simulink model "Linearization2"  (R2022a)
settings: Solver=VariableStepAuto  StartTime=0.0  StopTime=10.0  RelTol=1e-3
undefined symbols (not defined in the file): Aactuator, ac, AeroCoeff, ControlAllocation, DUmax, DUmin, EngineTable, F, fcs, ft, g, hground, IC, kg, LandingGear, Light, LPmethod, m, MIL, Mode_deflection_aileron, Mode_deflection_elevator, Mode_deflection_rudder, Mode_deflection_TVC_y, Mode_deflection_TVC_z, N, Ninv_2nozzle, Ninv_no_nozzle, PIController, s, Sensor, slug, state0, sysID_DAQ, sysID_OBES, Umax_2nozzle, Umax_no_nozzle, Umin_2nozzle, Umin_no_nozzle, WMM2020
libraries: aerolibconvert2 x19, slpidlib x6, simulink x6, sharedutil x4, aerolibatmos2 x3, aerolibwind2 x3, aerolibbdyn x3, aerolibgravity2 x2, sharedtransform x1
(part 3 of 9)

== system Linearization2/F-16 Vehicle Systems Model/Vehicle/Aerodynamics ==
  note: TODO: 這全部源自PlantData(物理系統)，不用感測器
  note: TODO: 這攻角、速度 來自感測器、AeroData System
  note: X
      | Y
      | Z
      | L
      | M
      | N
  note: 攻角 $\alpha$ 限制 -20 ~ 90度
      | 側滑角 $\beta$ 限制 -30 ~ 30 度
      | 馬赫數限制 0.1 ~ 0.6 度
  fcs_cmd : Inport
  " SB (deg)" : Inport  Port=2
  In Bus Element7 : Inport  Port=3  PortName=EnvData  Element=Pressure
  In Bus Element8 : Inport  Port=3  PortName=EnvData  Element=AirDensity
  In Bus Element9 : Inport  Port=3  PortName=EnvData  Element=qbar
  In Bus Element : Inport  Port=4  PortName=PlantData  Element=p
  In Bus Element1 : Inport  Port=4  PortName=PlantData  Element=q
  In Bus Element2 : Inport  Port=4  PortName=PlantData  Element=r
  In Bus Element3 : Inport  Port=4  PortName=PlantData  Element=alpha
  In Bus Element10 : Inport  Port=4  PortName=PlantData  Element=alpha
  In Bus Element4 : Inport  Port=4  PortName=PlantData  Element=beta
  In Bus Element6 : Inport  Port=4  PortName=PlantData  Element=Vt
  In Bus Element5 : Inport  Port=4  PortName=PlantData  Element=Vt
  Aerofynamic Coefficients : Subsystem
  AirframeActuators (no roll off) : Subsystem
  Angle Conversion1 : aerolibconvert2/Angle Conversion  IU=rad  OU=deg
  Angle Conversion2 : aerolibconvert2/Angle Conversion  IU=rad  OU=deg
  Angle Conversion3 : aerolibconvert2/Angle Conversion  Commented=on  IU=rad  OU=deg
  Bus Creator : BusCreator  Inputs=7
  Bus Selector : BusSelector  OutputSignals=right Aileron_deg,left Aileron_deg,right Elevator_deg,left Elevator_deg,Rudder_deg,LEF_deg
  Bus Selector1 : BusSelector  OutputSignals=right Aileron_deg,left Aileron_deg,right Elevator_deg,left Elevator_deg,Rudder_deg,LEF_deg
  Bus Selector2 : BusSelector  Commented=on  OutputSignals=LEF_deg
  Cbar(ft)1 : Constant  Value=ac.cbar
  Goto2 : Goto  Commented=on  GotoTag=LEF_deg
  Ground : Ground
  Leading Edge Flap : Subsystem  Commented=on
  Mux1 : Mux  Inputs=3
  Mux2 : Mux
  Product{6,9..14} (7 alike) : Product
  Sref(ft^2) : Constant  Value=ac.S
  Terminator{,1..3} (4 alike) : Terminator
  Velocity Conversion : aerolibconvert2/Velocity Conversion  Commented=on  IU=ft/s  OU=m/s
  b(ft)1 : Constant  Value=ac.b
  FM : Outport
  Bus Element Out : Outport  Port=2  PortName=ActSensor_Out
  wires:
  " SB (deg)"/1 -> Aerofynamic Coefficients/9(SB (deg)), Bus Creator/7  "SB_deg"
  In Bus Element1/1 -> Aerofynamic Coefficients/12(q)
  In Bus Element/1 -> Aerofynamic Coefficients/11(p)
  Angle Conversion2/1 -> Aerofynamic Coefficients/2(beta (deg))
  Angle Conversion1/1 -> Aerofynamic Coefficients/1(alpha (deg))
  In Bus Element2/1 -> Aerofynamic Coefficients/13(r)
  Ground/1 -> Aerofynamic Coefficients/15(h_AGL), Aerofynamic Coefficients/14(GearAngle)
  Mux1/1 -> Product9/2
  [qbar_S] -> Product9/1
  Aerofynamic Coefficients/6(Cn_T) -> Product14/2
  Aerofynamic Coefficients/5(Cm_T) -> Product12/2
  [qbar_S_cbar] -> Product12/1  "qbar_S_cbar"
  Aerofynamic Coefficients/4(Cl_T) -> Product13/2
  [qbar_S_b] -> Product13/1, Product14/1  "qbar_S_b"
  Aerofynamic Coefficients/1(CX_T) -> Mux1/1
  Aerofynamic Coefficients/2(CY_T) -> Mux1/2
  Aerofynamic Coefficients/3(CZ_T) -> Mux1/3
  Product13/1 -> Mux2/2
  Product12/1 -> Mux2/3
  Product14/1 -> Mux2/4
  Product9/1 -> Mux2/1
  Mux2/1 -> FM/1
  Sref(ft^2)/1 -> Product6/2
  b(ft)1/1 -> Product11/2  "b"
  Product11/1 -> [qbar_S_b]
  Product10/1 -> [qbar_S_cbar]
  Cbar(ft)1/1 -> Product10/2  "cbar"
  In Bus Element9/1 -> Product6/1  "qbar"
  Product6/1 -> Product11/1, Product10/1, [qbar_S]  "qbar_S"
  Leading Edge Flap/2(ActPositions) -> Goto2/1
  Velocity Conversion/1 -> Leading Edge Flap/1(vt (m/s))  "vt (m/s)"
  In Bus Element6/1 -> Aerofynamic Coefficients/10(vt (ft/s))
  In Bus Element8/1 -> Terminator1/1
  In Bus Element7/1 -> Terminator2/1
  AirframeActuators (no roll off)/1(ActPositions) -> Bus Selector/1
  fcs_cmd/1 -> AirframeActuators (no roll off)/1(fcs_cmd)
  In Bus Element3/1 -> Angle Conversion1/1
  In Bus Element4/1 -> Angle Conversion2/1
  In Bus Element5/1 -> Terminator/1  "vt (ft/s)"
  AirframeActuators (no roll off)/2(ActSensor_Out) -> Bus Selector1/1
  Bus Creator/1 -> Bus Element Out/1
  In Bus Element10/1 -> Terminator3/1
  Angle Conversion3/1 -> Leading Edge Flap/4(alpha (deg))
  Leading Edge Flap/1(ActSensor_Out) -> Bus Selector2/1
  Bus Selector1/1 -> Bus Creator/1  "<right Aileron_deg>"
  Bus Selector1/2 -> Bus Creator/2  "<left Aileron_deg>"
  Bus Selector1/3 -> Bus Creator/3  "<right Elevator_deg>"
  Bus Selector1/4 -> Bus Creator/4  "<left Elevator_deg>"
  Bus Selector1/5 -> Bus Creator/5  "<Rudder_deg>"
  Bus Selector1/6 -> Bus Creator/6  "<LEF_deg>"
  Bus Selector/1 -> Aerofynamic Coefficients/3(right alieron (deg))  "<right Aileron_deg>"
  Bus Selector/2 -> Aerofynamic Coefficients/4(left aileron (deg))  "<left Aileron_deg>"
  Bus Selector/3 -> Aerofynamic Coefficients/5(right elevator (deg))  "<right Elevator_deg>"
  Bus Selector/4 -> Aerofynamic Coefficients/6(left elevator (deg))  "<left Elevator_deg>"
  Bus Selector/5 -> Aerofynamic Coefficients/7(rudder (deg))  "<Rudder_deg>"
  Bus Selector/6 -> Aerofynamic Coefficients/8(LEF (deg))  "<LEF_deg>"

== system Linearization2/F-16 Vehicle Systems Model/Vehicle/Gravity Force ==
  note: 轉成行向量(column vector)
  note: 註：重力不會對飛機產生力矩，
      | 因為重力永遠作用在飛機重心上，
      | 力臂=0，所以力矩=0
  DCM_be : Inport
  In Bus Element : Inport  Port=2  PortName=EnvData  Element=g
  Gravity in Earth Axis : Gain  Gain=ac.m
  Reshape : Reshape  OutputDimensionality=Column vector (2-D)
  To Body Axes : Product  Multiplication=Matrix(*)
  Fgrav : Outport
  wires:
  In Bus Element/1 -> Gravity in Earth Axis/1
  To Body Axes/1 -> Fgrav/1
  DCM_be/1 -> To Body Axes/1
  Gravity in Earth Axis/1 -> Reshape/1
  Reshape/1 -> To Body Axes/2

== system Linearization2/F-16 Vehicle Systems Model/Vehicle/LandingGear GroundReaction ==
  note: 定義：
      | 慣性座標+Z軸朝上
      | 體座標+Z軸朝下
  note: 詹庭宇:
      | 此起落架模組源自MATLAB Simulink Example:HL-20
      | 我有做
      | 1.正負號的訂正
      | 2.拿掉/忽略輪胎側向力
  note: 詹庭宇:拿掉/忽略輪胎側向力模型，Fy=0
  LG_cmd : Inport
  In Bus Element4 : Inport  Port=2  PortName=EnvData  Element=hground
  In Bus Element5 : Inport  Port=2  PortName=EnvData  Element=hground
  In Bus Element6 : Inport  Port=2  PortName=EnvData  Element=hground
  In Bus Element3 : Inport  Port=3  PortName=PlantData
  In Bus Element1 : Inport  Port=3  PortName=PlantData
  In Bus Element2 : Inport  Port=3  PortName=PlantData
  Enable : EnablePort
  Demux : Demux  Outputs=3
  L Main Gear Geometry Forces and Moments : Subsystem  TreatAsAtomicUnit=on
  LeftMain : Selector  NumberOfDimensions=2  InputPortWidth=3  IndexOptions=Select all,Index vector (dialog)  Indices=-1,1  OutputSizes=1
  Nose : Selector  NumberOfDimensions=2  InputPortWidth=3  IndexOptions=Select all,Index vector (dialog)  Indices=-1,3  OutputSizes=1
  Nose Gear Geometry Forces and Moments : Subsystem  TreatAsAtomicUnit=on
  Pos_full_extend_ft Rows are X,Y,Z;cols are Left,Right,Nose gear Measured from CG in fts : Constant  Value=[-1.8405,-1.8405,9.9132 ; -3.8753,3.8753,0 ; 5.9161,5.9161, 6.2905]
  R Main Gear Geometry Forces and Moments : Subsystem  TreatAsAtomicUnit=on
  RightMain : Selector  NumberOfDimensions=2  InputPortWidth=3  IndexOptions=Select all,Index vector (dialog)  Indices=-1,2  OutputSizes=1
  Sum2 : Sum  Inputs=+++  InputSameDT=on  SaturateOnIntegerOverflow=on  OutDataTypeStr=Inherit: Same as first input
  FM : Outport
  Out Bus Element3 : Outport  Port=2  VectorParamsAs1DForOutWhenUnconnected=off  PortName=LGData  Element=Nose_WOW
  Out Bus Element4 : Outport  Port=2  VectorParamsAs1DForOutWhenUnconnected=off  PortName=LGData  Element=Nose_GearCmprs
  Out Bus Element5 : Outport  Port=2  VectorParamsAs1DForOutWhenUnconnected=off  PortName=LGData  Element=Nose_LG_down
  Out Bus Element6 : Outport  Port=2  VectorParamsAs1DForOutWhenUnconnected=off  PortName=LGData  Element=LeftMain_WOW
  Out Bus Element7 : Outport  Port=2  VectorParamsAs1DForOutWhenUnconnected=off  PortName=LGData  Element=LeftMain_GearCmprs
  Out Bus Element8 : Outport  Port=2  VectorParamsAs1DForOutWhenUnconnected=off  PortName=LGData  Element=LeftMain_LG_down
  Out Bus Element9 : Outport  Port=2  VectorParamsAs1DForOutWhenUnconnected=off  PortName=LGData  Element=RightMain_WOW
  Out Bus Element10 : Outport  Port=2  VectorParamsAs1DForOutWhenUnconnected=off  PortName=LGData  Element=RightMain_GearCmprs
  Out Bus Element11 : Outport  Port=2  VectorParamsAs1DForOutWhenUnconnected=off  PortName=LGData  Element=RightMain_LG_down
  wires:
  In Bus Element4/1 -> L Main Gear Geometry Forces and Moments/1(ground_z_ft)
  In Bus Element3/1 -> L Main Gear Geometry Forces and Moments/2(plant)
  In Bus Element1/1 -> R Main Gear Geometry Forces and Moments/2(plant)
  In Bus Element2/1 -> Nose Gear Geometry Forces and Moments/2(plant)
  R Main Gear Geometry Forces and Moments/1(FM) -> Sum2/2
  L Main Gear Geometry Forces and Moments/1(FM) -> Sum2/1
  R Main Gear Geometry Forces and Moments/3(GearCmprs) -> Out Bus Element10/1
  R Main Gear Geometry Forces and Moments/2(WOW) -> Out Bus Element9/1
  L Main Gear Geometry Forces and Moments/2(WOW) -> Out Bus Element6/1
  L Main Gear Geometry Forces and Moments/3(GearCmprs) -> Out Bus Element7/1
  RightMain/1 -> R Main Gear Geometry Forces and Moments/3(GearLoc)
  Nose/1 -> Nose Gear Geometry Forces and Moments/3(GearLoc)
  Pos_full_extend_ft Rows are X,Y,Z;cols are Left,Right,Nose gear Measured from CG in fts/1 -> LeftMain/1, Nose/1, RightMain/1
  Nose Gear Geometry Forces and Moments/1(FM) -> Sum2/3
  Nose Gear Geometry Forces and Moments/2(WOW) -> Out Bus Element3/1
  Nose Gear Geometry Forces and Moments/3(GearCmprs) -> Out Bus Element4/1
  Sum2/1 -> FM/1
  LeftMain/1 -> L Main Gear Geometry Forces and Moments/3(GearLoc)
  LG_cmd/1 -> Demux/1
  Demux/1 -> Out Bus Element5/1
  Demux/2 -> Out Bus Element11/1
  Demux/3 -> Out Bus Element8/1
  In Bus Element5/1 -> R Main Gear Geometry Forces and Moments/1(ground_z_ft)
  In Bus Element6/1 -> Nose Gear Geometry Forces and Moments/1(ground_z_ft)

== system Linearization2/F-16 Vehicle Systems Model/Vehicle/Propulsion ==
  note: 繞"固定座標旋轉"旋轉(外在旋轉extrinsic rotation)
  note: Thrust Vector Nozzle Module 向量噴嘴模組
  note: Commands_TVC_rY_pitch_deg
      | Commands_TVC_rZ_yaw_deg
      | Commands_TVC_lY_pitch_deg
      | Commands_TVC_lZ_yaw_deg
  note: Inlet 進氣道
  note: 高度限制 0 ~ 50000 ft
      | 馬赫數限制 0 ~ 1 馬赫
  Bus Element In2 : Inport  PortName=fadec_cmd
  In Bus Element3 : Inport  PortName=fadec_cmd  Element=thrust
  In Bus Element1 : Inport  Port=2  PortName=EnvData  Element=Mach
  Bus Element In1 : Inport  Port=3  PortName=PlantData  Element=beta
  Bus Element In : Inport  Port=3  PortName=PlantData  Element=alpha
  In Bus Element : Inport  Port=3  PortName=PlantData  Element=altitude
  Actuators : Subsystem
  Afterburning Turbofan Jet Engine : Subsystem
  Cos : Trigonometry  Operator=cos
  Cos1 : Trigonometry  Operator=cos
  Gain1 : Gain  Gain=0.5
  IC1 : InitialCondition  Commented=through  Value=IC.thrust_lbf
  Product : Product  Inputs=3
  Thrust Vector Nozzle ZY1 : Subsystem
  nozzle position1 : Constant  Value=ac.lt1
  nozzle position2 : Constant  Value=ac.mt
  r2d1 : Gain  Gain=-1  SaturateOnIntegerOverflow=on  OutDataTypeStr=Inherit: Same as input  ParamDataTypeStr=Inherit: Same as input
  FM : Outport
  Bus Element Out : Outport  Port=2  PortName=ActSensor_Out
  Bus Element Out1 : Outport  Port=3  PortName=PropData  Element=Tx
  Bus Element Out2 : Outport  Port=3  PortName=PropData  Element=Ty
  Bus Element Out3 : Outport  Port=3  PortName=PropData  Element=Tz
  Bus Element Out4 : Outport  Port=3  PortName=PropData  Element=T
  Bus Element Out5 : Outport  Port=3  PortName=PropData  Element=engine_state
  wires:
  Actuators/2(ActSensor_Out) -> Bus Element Out/1
  nozzle position1/1 -> Thrust Vector Nozzle ZY1/3(" lt1")
  Actuators/1(ActPositions) -> Thrust Vector Nozzle ZY1/2(Actuator (deg))
  Thrust Vector Nozzle ZY1/1(FM) -> FM/1
  Product/1 -> Afterburning Turbofan Jet Engine/1(Mach)
  r2d1/1 -> Afterburning Turbofan Jet Engine/2(H (ft))
  Cos/1 -> Product/2
  Bus Element In1/1 -> Cos1/1  "beta (rad)"
  In Bus Element1/1 -> Product/1
  Cos1/1 -> Product/3
  Bus Element In/1 -> Cos/1  "alpha (rad)"
  In Bus Element/1 -> r2d1/1
  Bus Element In2/1 -> Actuators/1(Commands)
  Thrust Vector Nozzle ZY1/2(Tx) -> Bus Element Out1/1
  Thrust Vector Nozzle ZY1/3(Ty) -> Bus Element Out2/1
  Thrust Vector Nozzle ZY1/4(Tz) -> Bus Element Out3/1
  nozzle position2/1 -> Thrust Vector Nozzle ZY1/4(" mt")
  IC1/1 -> Gain1/1, Bus Element Out4/1  "thrust"
  Afterburning Turbofan Jet Engine/1(T (lbf)) -> IC1/1  "thrust"
  Afterburning Turbofan Jet Engine/2(engine_state) -> Bus Element Out5/1
  In Bus Element3/1 -> Afterburning Turbofan Jet Engine/3(Tc (lbf))  "Commands_Tc"
  Gain1/1 -> Thrust Vector Nozzle ZY1/1(T1)  "thrust"

== system Linearization2/F-16 Vehicle Systems Model/Vehicle/Propulsion(two_nozzles) ==
  note: Thrust Vector Nozzle Module 向量噴嘴模組
  note: Commands_TVC_ry_pitch_deg
      | Commands_TVC_rz_yaw_deg
      | Commands_TVC_ly_pitch_deg
      | Commands_TVC_lz_yaw_deg
  note: Inlet 進氣道
  note: 高度限制 0 ~ 50000 ft
      | 馬赫數限制 0 ~ 1 馬赫
  Bus Element In2 : Inport  PortName=fadec_cmd
  In Bus Element3 : Inport  PortName=fadec_cmd  Element=thrust
  In Bus Element1 : Inport  Port=2  PortName=EnvData  Element=Mach
  Bus Element In1 : Inport  Port=3  PortName=PlantData  Element=beta
  Bus Element In : Inport  Port=3  PortName=PlantData  Element=alpha
  In Bus Element : Inport  Port=3  PortName=PlantData  Element=altitude
  Actuators : Subsystem
  Actuators1 : Subsystem
  Add{,1..5} (6 alike) : Sum
  Afterburning Turbofan Jet Engine : Subsystem
  Bus Creator : BusCreator  Inputs=4
  Cos : Trigonometry  Operator=cos
  Cos1 : Trigonometry  Operator=cos
  Gain1 : Gain  Gain=0.5
  IC1 : InitialCondition  Commented=through  Value=IC.thrust_lbf
  Mux2 : Mux  Inputs=6
  Product : Product  Inputs=3
  Thrust Vector Nozzle ZY1 : Subsystem
  Thrust Vector Nozzle ZY2 : Subsystem
  nozzle position1 : Constant  Value=ac.lt1
  nozzle position2 : Constant  Value=ac.mt
  nozzle position3 : Constant  Value=ac.lt1
  nozzle position4 : Constant  Value=ac.mt
  r2d1 : Gain  Gain=-1  SaturateOnIntegerOverflow=on  OutDataTypeStr=Inherit: Same as input  ParamDataTypeStr=Inherit: Same as input
  FM : Outport
  Bus Element Out : Outport  Port=2  PortName=ActSensor_Out
  Bus Element Out4 : Outport  Port=3  PortName=PropData  Element=T
  Bus Element Out5 : Outport  Port=3  PortName=PropData  Element=engine_state
  Bus Element Out15 : Outport  Port=3  PortName=PropData  Element=Tx
  Bus Element Out16 : Outport  Port=3  PortName=PropData  Element=Ty
  Bus Element Out17 : Outport  Port=3  PortName=PropData  Element=Tz
  wires:
  nozzle position1/1 -> Thrust Vector Nozzle ZY1/3(" lt1")
  Actuators/1(ActPositions) -> Thrust Vector Nozzle ZY1/2(Actuator (deg))
  Product/1 -> Afterburning Turbofan Jet Engine/1(Mach)
  r2d1/1 -> Afterburning Turbofan Jet Engine/2(H (ft))
  Cos/1 -> Product/2
  Bus Element In1/1 -> Cos1/1  "beta (rad)"
  In Bus Element1/1 -> Product/1
  Cos1/1 -> Product/3
  Bus Element In/1 -> Cos/1  "alpha (rad)"
  In Bus Element/1 -> r2d1/1
  Bus Element In2/1 -> Actuators/1(Commands), Actuators1/1(Commands)
  Thrust Vector Nozzle ZY1/1(Trx) -> Add/1
  Thrust Vector Nozzle ZY1/2(Try) -> Add1/1
  Thrust Vector Nozzle ZY1/3(Trz) -> Add2/1
  nozzle position2/1 -> Thrust Vector Nozzle ZY1/4(" mt")
  IC1/1 -> Gain1/1, Bus Element Out4/1  "thrust"
  Afterburning Turbofan Jet Engine/1(T (lbf)) -> IC1/1  "thrust"
  Afterburning Turbofan Jet Engine/2(engine_state) -> Bus Element Out5/1
  In Bus Element3/1 -> Afterburning Turbofan Jet Engine/3(Tc (lbf))  "Commands_Tc"
  Gain1/1 -> Thrust Vector Nozzle ZY1/1(T1), Thrust Vector Nozzle ZY2/1(T1)  "thrust"
  Thrust Vector Nozzle ZY1/4(Mrx) -> Add3/1
  Thrust Vector Nozzle ZY1/5(Mry) -> Add4/1
  Thrust Vector Nozzle ZY1/6(Mrz) -> Add5/1
  nozzle position3/1 -> Thrust Vector Nozzle ZY2/3(" lt1")
  nozzle position4/1 -> Thrust Vector Nozzle ZY2/4(" mt")
  Actuators1/1(ActPositions) -> Thrust Vector Nozzle ZY2/2(Actuator (deg))
  Thrust Vector Nozzle ZY2/1(Tlx) -> Add/2
  Thrust Vector Nozzle ZY2/2(Tly) -> Add1/2
  Thrust Vector Nozzle ZY2/3(Tlz) -> Add2/2
  Thrust Vector Nozzle ZY2/4(Mlx) -> Add3/2
  Thrust Vector Nozzle ZY2/5(Mly) -> Add4/2
  Thrust Vector Nozzle ZY2/6(Mlz) -> Add5/2
  Bus Creator/1 -> Bus Element Out/1
  Add/1 -> Mux2/1, Bus Element Out15/1
  Add1/1 -> Mux2/2, Bus Element Out16/1
  Add2/1 -> Mux2/3, Bus Element Out17/1
  Add3/1 -> Mux2/4
  Add4/1 -> Mux2/5
  Add5/1 -> Mux2/6
  Mux2/1 -> FM/1
  Actuators/2(ActSensor_Out.TVC_ry_pitch_deg) -> Bus Creator/1  "TVC_ry_pitch_deg"
  Actuators/3(ActSensor_Out.TVC_rz_yaw_deg) -> Bus Creator/2  "TVC_rz_yaw_deg"
  Actuators1/2(ActSensor_Out.TVC_ly_pitch_deg) -> Bus Creator/3  "TVC_ly_pitch_deg"
  Actuators1/3(ActSensor_Out.TVC_lz_yaw_deg) -> Bus Creator/4  "TVC_lz_yaw_deg"

== system Linearization2/F-16 Vehicle Systems Model/pqr NDI Controller/Control Allocation ==
  IN_MAT1 : Inport
  Input : Inport  Port=2
  Input1 : Inport  Port=3
  Input2 : Inport  Port=4
  y_bar : Inport  Port=5
  g1 : Inport  Port=6
  N : Inport  Port=7
  Abs : Abs  SaturateOnIntegerOverflow=off
  Abs1 : Abs  SaturateOnIntegerOverflow=off
  Abs2 : Abs  SaturateOnIntegerOverflow=off
  Angle Conversion : aerolibconvert2/Angle Conversion  IU=rad  OU=deg
  CGIwrap : Subsystem  TreatAsAtomicUnit=on
  CGIwrap1 : Subsystem  TreatAsAtomicUnit=on
  Chart : Stateflow chart  TreatAsAtomicUnit=on  SystemSampleTime=fcs.Ts
      settings: PortSchema="{\"entries\":[{\"content\":{\"sides\":[{\"content\":{\"connectorIds\":[\"In6\",\"In1\",\"In2\",\"In4\",\"In3\",\"In5\"]},\"type\":\"ConnectorPlacement.EquallySpacedRectSide\",\"uuid\":\"6d076ae3-a9f2-4680-9177-aea4e2fc761d\"},{\"content\":{\"connectorIds\":[\"Out1\"],\"side\":\"RIGHT\"},\"type\":\"ConnectorPlacement.EquallySpacedRectSide\",\"uuid\":\"02bbf86f-ce68-419e-b070-bdc8bcbcb5dc\"},{\"content\":{\"connectorIds\":[],\"side\":\"TOP\"},\"type\":\"ConnectorPlacement.EquallySpacedRectSide\",\"uuid\":\"3dbba490-ab37-41e3-b3e5-776a7fc0e7cf\"}]},\"type\":\"ConnectorPlacement.EquallySpacedConnector\",\"uuid\":\"e8ffa1d9-13bd-4b1f-b66c-de77a24e235e\"}],\"packageUris\":[\"http://schema.mathworks.com/mf0/Connector/19700101\"],\"version\":\"1.0\"}"
  Constant : Constant  Value=0
  ControlAllocation : Constant  Value=ControlAllocation
  DAISY_CHAINING : Subsystem  TreatAsAtomicUnit=on
  DA_Allocation : Subsystem  TreatAsAtomicUnit=on
  Discrete Derivative : simulink/Discrete/Discrete Derivative  gainval=1.0  ICPrevScaledInput=0.0  OutMin=[]  OutMax=[]  OutDataType=fixdt(1, 16)  OutScaling=2^-10  DoSatur=off
  Discrete Derivative1 : simulink/Discrete/Discrete Derivative  gainval=1.0  ICPrevScaledInput=0.0  OutMin=[]  OutMax=[]  OutDataType=fixdt(1, 16)  OutScaling=2^-10  DoSatur=off
  IC : InitialCondition  Value=0
  IC1 : InitialCondition  Value=0
  IC2 : InitialCondition  Value=[0 0 0 0 0 0 0 0 0]
  If : If  IfExpression=u1 == 1  ElseIfExpressions=u1 == 2,u1 == 3,u1 == 4,u1 == 5,u1==6,u1==7,u1==8,u1==9,u1==10
  LPwrap_def1 : Subsystem  TreatAsAtomicUnit=on
  LPwrap_lift : Subsystem  TreatAsAtomicUnit=on
  LPwrap_sig : Subsystem  TreatAsAtomicUnit=on
  LPwrap_thrust : Subsystem  TreatAsAtomicUnit=on
  Manual Switch : ManualSwitch  CurrentSetting=0
  Merge1 : Merge  Inputs=11
  Pseudo_inverses_ShunYuanChang2019 : Subsystem  TreatAsAtomicUnit=on
  To Workspace : ToWorkspace  VariableName=u  SaveFormat=Timeseries  SampleTime=-1
  To Workspace1 : ToWorkspace  VariableName=altitude_dot  SaveFormat=Timeseries  SampleTime=-1
  To Workspace2 : ToWorkspace  VariableName=Vt_dot  SaveFormat=Timeseries  SampleTime=-1
  Weighted_Pseudo_inverses : Subsystem  TreatAsAtomicUnit=on
  control_management : Subsystem  TreatAsAtomicUnit=on
  Du : Outport
  wires:
  If/1 -> Weighted_Pseudo_inverses/Action
  DAISY_CHAINING/1(Out1) -> Merge1/2
  If/2 -> DAISY_CHAINING/Action
  Weighted_Pseudo_inverses/1(Out1) -> Merge1/1
  IN_MAT1/1 -> control_management/1(IN_MAT), DA_Allocation/1(IN_MAT), CGIwrap/1(IN_MAT), Weighted_Pseudo_inverses/1(IN_MAT), DAISY_CHAINING/1(IN_MAT), LPwrap_lift/1(IN_MAT), LPwrap_sig/1(IN_MAT), LPwrap_thrust/1(IN_MAT), CGIwrap1/1(IN_MAT), LPwrap_def1/1(IN_MAT)
  Chart/1(CA) -> Manual Switch/1
  ControlAllocation/1 -> Manual Switch/2
  If/6 -> LPwrap_def1/Action
  If/7 -> LPwrap_lift/Action
  If/8 -> LPwrap_sig/Action
  If/9 -> LPwrap_thrust/Action
  LPwrap_lift/1(Out1) -> Merge1/7
  LPwrap_sig/1(Out1) -> Merge1/8
  LPwrap_thrust/1(Out1) -> Merge1/9
  Input/1 -> Angle Conversion/1
  Angle Conversion/1 -> Chart/1(alpha)
  Input2/1 -> Abs/1
  Abs/1 -> Chart/3(altitude), Discrete Derivative1/1
  Discrete Derivative/1 -> Abs1/1
  Discrete Derivative1/1 -> Abs2/1
  Input1/1 -> Chart/2(Vt), Discrete Derivative/1
  IC/1 -> Chart/5(altitude_dot), To Workspace1/1
  Abs2/1 -> IC/1
  Abs1/1 -> IC1/1
  IC1/1 -> Chart/4(Vt_dot), To Workspace2/1
  If/10 -> Pseudo_inverses_ShunYuanChang2019/Action
  Pseudo_inverses_ShunYuanChang2019/1(Output) -> Merge1/10
  y_bar/1 -> Pseudo_inverses_ShunYuanChang2019/1(y_bar)
  g1/1 -> Pseudo_inverses_ShunYuanChang2019/2(g1)
  N/1 -> Pseudo_inverses_ShunYuanChang2019/3(N)
  Constant/1 -> Chart/6(switchhh)
  LPwrap_def1/1(Out1) -> Merge1/6
  IC2/1 -> Du/1
  Merge1/1 -> IC2/1
  control_management/1(Out1) -> Merge1/5
  Manual Switch/1 -> If/1, To Workspace/1
  CGIwrap1/1(Out1) -> Merge1/11
  DA_Allocation/1(Out1) -> Merge1/4
  CGIwrap/1(Out1) -> Merge1/3
  If/3 -> CGIwrap/Action
  If/4 -> DA_Allocation/Action
  If/5 -> control_management/Action
  If/11 -> CGIwrap1/Action

== system Linearization2/F-16 Vehicle Systems Model/pqr NDI Controller/MakeINMAT ==
  note: 飛控系統的取樣時間(秒)
  note: 控制配置的權重矩陣 $N^{-1}$
      | (定義於 PreLoadFcn.m)
  note: 下標1表示在列後面擴增
      | 下標2表示在行後面擴增
  f1 : Inport
  g1 : Inport  Port=2
  In3 : Inport  Port=3
  Constant : Constant  Value=LPmethod
  Constant1 : Constant  Value=[0;0;0;0]
  Constant10 : Constant  Value=Umin_no_nozzle
  Constant2 : Constant  Value=Umax_2nozzle
  Constant3 : Constant  Value=Umin_2nozzle
  Constant4 : Constant  Value=[1 1 1 1 1 1 1 1 1]
  Constant5 : Constant  Value=fcs.Ts
  Constant6 : Constant  Value=DUmax
  Constant7 : Constant  Value=[0;0;0;0;0;0;0;0;0]
  Constant8 : Constant  Value=DUmin
  Constant9 : Constant  Value=Umax_no_nozzle
  Manual Switch : ManualSwitch
  Manual Switch1 : ManualSwitch
  Manual Switch2 : ManualSwitch
  Matrix Concatenate{,2,4,6} (4 alike) : Concatenate  Mode=Multidimensional array  ConcatenateDimension=2
  Matrix Concatenate1 : Concatenate  Mode=Multidimensional array
  Matrix Concatenate3 : Concatenate  NumInputs=5  Mode=Multidimensional array
  Matrix Concatenate5 : Concatenate  NumInputs=4  Mode=Multidimensional array
  Signal Specification : SignalSpecification  Dimensions=[3 1]
  Signal Specification{1..2,4..9} (8 alike) : SignalSpecification  Dimensions=[1,9]
  Signal Specification3 : SignalSpecification  Dimensions=[3 9]
  To Workspace2 : ToWorkspace  VariableName=B_matrix  SaveFormat=Timeseries  SampleTime=-1
  inverse of weighting matrix N : Constant  Value=Ninv_2nozzle
  inverse of weighting matrix N1 : Constant  Value=Ninv_no_nozzle
  IN_MAT : Outport
  wires:
  Matrix Concatenate6/1 -> Matrix Concatenate5/4
  Matrix Concatenate3/1 -> Matrix Concatenate4/1
  Signal Specification3/1 -> Matrix Concatenate/1
  Manual Switch1/1 -> Matrix Concatenate3/2
  Matrix Concatenate4/1 -> Matrix Concatenate5/3
  Matrix Concatenate/1 -> Matrix Concatenate5/1
  Signal Specification/1 -> Matrix Concatenate/2
  Manual Switch/1 -> Matrix Concatenate3/1
  Matrix Concatenate5/1 -> IN_MAT/1
  f1/1 -> Signal Specification/1
  g1/1 -> To Workspace2/1, Signal Specification3/1
  Constant4/1 -> Signal Specification4/1
  Signal Specification4/1 -> Matrix Concatenate3/5
  Constant1/1 -> Matrix Concatenate1/1
  Constant/1 -> Matrix Concatenate1/2
  Matrix Concatenate1/1 -> Matrix Concatenate4/2
  In3/1 -> Signal Specification5/1
  Signal Specification5/1 -> Matrix Concatenate2/1
  Constant5/1 -> Matrix Concatenate2/2
  Matrix Concatenate2/1 -> Matrix Concatenate5/2
  Signal Specification6/1 -> Matrix Concatenate3/3
  Signal Specification7/1 -> Matrix Concatenate3/4
  Constant6/1 -> Signal Specification6/1  "Umax"
  Constant8/1 -> Signal Specification7/1  "Umax"
  Constant3/1 -> Signal Specification2/1  "Umin"
  Constant2/1 -> Signal Specification1/1  "Umax"
  Signal Specification1/1 -> Manual Switch/1
  Signal Specification2/1 -> Manual Switch1/1
  Signal Specification8/1 -> Manual Switch/2
  Constant9/1 -> Signal Specification8/1  "Umax"
  Signal Specification9/1 -> Manual Switch1/2
  Constant10/1 -> Signal Specification9/1  "Umin"
  Constant7/1 -> Matrix Concatenate6/2
  inverse of weighting matrix N/1 -> Manual Switch2/1
  inverse of weighting matrix N1/1 -> Manual Switch2/2
  Manual Switch2/1 -> Matrix Concatenate6/1

== system Linearization2/F-16 Vehicle Systems Model/pqr NDI Controller/Mode_deflection ==
  note: 偏轉模式： 0=傳統左右副翼差動
      | 1=左右副翼獨立偏轉
      | 其它=左右副翼獨立偏轉
  note: 偏轉模式： 0=傳統左右升降舵同動
      | 1=左右升降舵獨立偏轉
      | 其它=左右升降舵獨立偏轉
  note: 偏轉模式： 0=傳統左右方向舵同動
      | 1=左右方向舵獨立偏轉
      | 2=左右方向舵差動(產生減速效果)
      | 其它=左右方向舵獨立偏轉
  note: 偏轉模式： 0=傳統左右向量噴嘴固定不動
      | 1=左右向量噴嘴左右獨立偏轉
      | 2=左右向量噴嘴左右同動
      | 其它=左右向量噴嘴左右獨立偏轉
  note: 偏轉模式： 0=傳統左右向量噴嘴固定不動
      | 1=左右向量噴嘴上下獨立偏轉
      | 2=左右向量噴嘴上下同動(產生俯仰)
      | 3=左右向量噴嘴上下差動(產生滾轉)
      | 其它=左右向量噴嘴上下獨立偏轉
  dra : Inport
  dla : Inport  Port=2
  dre : Inport  Port=3
  dle : Inport  Port=4
  drr : Inport  Port=5
  dlr : Inport  Port=6
  dry : Inport  Port=7
  drz : Inport  Port=8
  dly : Inport  Port=9
  dlz : Inport  Port=10
  Constant{,3,7,10} (4 alike) : Constant  Value=0
  Constant1 : Constant  Value=Mode_deflection_aileron
  Constant2 : Constant  Value=Mode_deflection_elevator
  Constant4 : Constant  Value=Mode_deflection_TVC_y
  Constant5 : Constant  Value=Mode_deflection_rudder
  Constant6 : Constant  Value=Mode_deflection_TVC_y
  Constant8 : Constant  Value=Mode_deflection_TVC_z
  Constant9 : Constant  Value=Mode_deflection_TVC_z
  Gain : Gain  Gain=-1
  Gain1 : Gain  Gain=-1
  Gain2 : Gain  Gain=-1
  Multiport Switch : MultiPortSwitch  DataPortOrder=Zero-based contiguous  Inputs=2  zeroidx=on  SaturateOnIntegerOverflow=off  InputSameDT=off
  Multiport Switch1 : MultiPortSwitch  DataPortOrder=Zero-based contiguous  Inputs=2  zeroidx=on  SaturateOnIntegerOverflow=off  InputSameDT=off
  Multiport Switch2 : MultiPortSwitch  DataPortOrder=Zero-based contiguous  DataPortForDefault=Additional data port  zeroidx=on  SaturateOnIntegerOverflow=off  InputSameDT=off
  Multiport Switch3 : MultiPortSwitch  DataPortOrder=Zero-based contiguous  Inputs=4  DataPortForDefault=Additional data port  zeroidx=on  SaturateOnIntegerOverflow=off  InputSameDT=off
  Multiport Switch4 : MultiPortSwitch  DataPortOrder=Zero-based contiguous  DataPortForDefault=Additional data port  zeroidx=on  SaturateOnIntegerOverflow=off  InputSameDT=off
  Multiport Switch5 : MultiPortSwitch  DataPortOrder=Zero-based contiguous  Inputs=4  DataPortForDefault=Additional data port  zeroidx=on  SaturateOnIntegerOverflow=off  InputSameDT=off
  Multiport Switch6 : MultiPortSwitch  DataPortOrder=Zero-based contiguous  DataPortForDefault=Additional data port  zeroidx=on  SaturateOnIntegerOverflow=off  InputSameDT=off
  right_aileron : Outport  VectorParamsAs1DForOutWhenUnconnected=off
  left_aileron : Outport  Port=2  VectorParamsAs1DForOutWhenUnconnected=off
  right_elevator : Outport  Port=3  VectorParamsAs1DForOutWhenUnconnected=off
  left_elevator : Outport  Port=4  VectorParamsAs1DForOutWhenUnconnected=off
  rudder : Outport  Port=5  VectorParamsAs1DForOutWhenUnconnected=off
  left_rudder : Outport  Port=6  VectorParamsAs1DForOutWhenUnconnected=off
  "TVC_ry " : Outport  Port=7  VectorParamsAs1DForOutWhenUnconnected=off
  TVC_rz : Outport  Port=8  VectorParamsAs1DForOutWhenUnconnected=off
  "TVC_ly " : Outport  Port=9  VectorParamsAs1DForOutWhenUnconnected=off
  "TVC_lz " : Outport  Port=10  VectorParamsAs1DForOutWhenUnconnected=off
  wires:
  Gain2/1 -> Multiport Switch3/5
  Gain1/1 -> Multiport Switch4/4
  Multiport Switch4/1 -> left_rudder/1
  Multiport Switch2/1 -> "TVC_lz "/1
  Constant3/1 -> Multiport Switch2/2
  drz/1 -> Multiport Switch6/3, Multiport Switch6/4, Multiport Switch6/5, Multiport Switch2/4
  Constant10/1 -> Multiport Switch6/2
  Multiport Switch6/1 -> TVC_rz/1
  Constant8/1 -> Multiport Switch2/1
  dlz/1 -> Multiport Switch2/3, Multiport Switch2/5
  Constant9/1 -> Multiport Switch6/1
  Multiport Switch5/1 -> "TVC_ry "/1
  Constant7/1 -> Multiport Switch5/2
  Constant6/1 -> Multiport Switch5/1
  Constant/1 -> Multiport Switch3/2
  dly/1 -> Multiport Switch3/6, Multiport Switch3/3
  Multiport Switch/1 -> left_aileron/1
  dre/1 -> right_elevator/1, Multiport Switch1/2
  dle/1 -> Multiport Switch1/3
  Multiport Switch1/1 -> left_elevator/1
  dla/1 -> Multiport Switch/3
  drr/1 -> Multiport Switch4/2, Gain1/1, rudder/1
  dry/1 -> Gain2/1, Multiport Switch3/4, Multiport Switch5/6, Multiport Switch5/5, Multiport Switch5/4, Multiport Switch5/3
  Constant5/1 -> Multiport Switch4/1
  dra/1 -> right_aileron/1, Gain/1
  Constant2/1 -> Multiport Switch1/1
  Constant4/1 -> Multiport Switch3/1
  Gain/1 -> Multiport Switch/2
  Constant1/1 -> Multiport Switch/1
  dlr/1 -> Multiport Switch4/3, Multiport Switch4/5
  Multiport Switch3/1 -> "TVC_ly "/1

== system Linearization2/F-16 Vehicle Systems Model/pqr NDI Controller/control matrix g1 ==
  note: m
      | ix
      | iy
      | iz
      | ixy
      | ixz
      | iyz
  note: 1  gp_dra1
      |     gp_dla1
      |     gp_dre1
      |     gp_dle1
      |     gp_dr1
      |     gp_dra2
      |     gp_dla2
      |     gp_dre2
      |     gp_dle2
      |     gp_dr2
      |
      | 11 gq_dra
      |      gq_dla
      |      gq_dre
      |      gq_dle
      |
      | 15 gr_dra1
      |      gr_dla1
      |      gr_dre1
      |      gr_dle1
      |      gr_dr1
      |      gr_dra2
      |      gr_dla2
      |      gr_dre2
      |      gr_dle2
      |      gr_dr2
  note: $g_1 {\left({\overset{-}{x} }_1 \right)}={\left[\begin{array}{ccccccccc} g_{p_{\delta_{ra} } } & g_{p_{\delta_{la} } } & g_{p_{\delta_{re} } } & g_{p_{\delta_{le} } } & g_{p_{\delta_r } } & g_{p_{\delta_{ry} } } & g_{p_{\delta_{rz} } } & g_{p_{\delta_{ly} } } & g_{p_{\delta_{lz} } } \\ g_{q_{\delta_{ra} } } & g_{q_{\delta_{la} } } & g_{q_{\delta_{re} } } & g_{q_{\delta_{le} } } & 0 & g_{q_{\delta_{ry} } } & 0 & g_{q_{\delta_{ly} } } & 0 \\ g_{r_{\delta_{ra} } } & g_{r_{\delta_{la} } } & g_{r_{\delta_{re} } } & g_{r_{\delta_{le} } } & g_{r_{\delta_r } } & g_{r_{\delta_{ry} } } & g_{r_{\delta_{rz} } } & g_{r_{\delta_{ly} } } & g_{r_{\delta_{lz} } } \end{array}\right]}$
  coef g : Inport
  Thrust T : Inport  Port=2
  Engine nozzle after of c.g.1 : Constant  Value=ac.lt1
  Engine nozzle after of c.g.2 : Constant  Value=ac.mt
  Gain : Gain  Gain=1/2
  Ix(slug*ft^2) : Constant  Value=ac.Ix
  Ixy(slug*ft^2) : Constant  Value=ac.Ixy
  Ixz(slug*ft^2) : Constant  Value=ac.Ixz
  Iy(slug*ft^2) : Constant  Value=ac.Iy
  Iyz(slug*ft^2) : Constant  Value=ac.Iyz
  Iz(slug*ft^2) : Constant  Value=ac.Iz
  Matrix Concatenate : Concatenate  NumInputs=3  Mode=Multidimensional array
  Mux : Mux  Inputs=7
  "Pitching " : Subsystem
  "Rolling " : Subsystem
  "Yawing " : Subsystem
  m(slugs) : Constant  Value=ac.m
  g1 : Outport  VectorParamsAs1DForOutWhenUnconnected=off
  wires:
  "Yawing "/1(g1 Row3) -> Matrix Concatenate/3
  "Pitching "/1(g1 Row2) -> Matrix Concatenate/2
  "Rolling "/1(g1 Row1) -> Matrix Concatenate/1
  Mux/1 -> "Rolling "/2(inertia), "Pitching "/2(inertia), "Yawing "/2(inertia)
  coef g/1 -> "Yawing "/1(control_g), "Pitching "/1(control_g), "Rolling "/1(control_g)
  Thrust T/1 -> Gain/1
  Engine nozzle after of c.g.1/1 -> "Yawing "/4("lt1 "), "Pitching "/4(lt1), "Rolling "/4(lt1)
  Iyz(slug*ft^2)/1 -> Mux/7
  Ix(slug*ft^2)/1 -> Mux/2
  Iy(slug*ft^2)/1 -> Mux/3
  Ixy(slug*ft^2)/1 -> Mux/5
  Ixz(slug*ft^2)/1 -> Mux/6
  Iz(slug*ft^2)/1 -> Mux/4
  m(slugs)/1 -> Mux/1
  Matrix Concatenate/1 -> g1/1
  Engine nozzle after of c.g.2/1 -> "Rolling "/5(mt), "Pitching "/5(mt), "Yawing "/5(mt)
  Gain/1 -> "Rolling "/3(Thrust), "Pitching "/3(Thrust), "Yawing "/3(Thrust)

== system Linearization2/F-16 Vehicle Systems Model/sysID_Onboard_Excitation_System/Mode_deflection ==
  note: 偏轉模式： 0=傳統左右副翼差動
      | 1=左右副翼獨立偏轉
      | 其它=左右副翼獨立偏轉
  note: 偏轉模式： 0=傳統左右升降舵同動
      | 1=左右升降舵獨立偏轉
      | 其它=左右升降舵獨立偏轉
  note: 偏轉模式： 0=傳統左右方向舵同動
      | 1=左右方向舵獨立偏轉
      | 2=左右方向舵差動(產生減速效果)
      | 其它=左右方向舵獨立偏轉
  note: 偏轉模式： 0=傳統左右向量噴嘴固定不動
      | 1=左右向量噴嘴左右獨立偏轉
      | 2=左右向量噴嘴左右同動
      | 其它=左右向量噴嘴左右獨立偏轉
  note: 偏轉模式： 0=傳統左右向量噴嘴固定不動
      | 1=左右向量噴嘴上下獨立偏轉
      | 2=左右向量噴嘴上下同動(產生俯仰)
      | 3=左右向量噴嘴上下差動(產生滾轉)
      | 其它=左右向量噴嘴上下獨立偏轉
  dra : Inport
  dla : Inport  Port=2
  dre : Inport  Port=3
  dle : Inport  Port=4
  drr : Inport  Port=5
  dlr : Inport  Port=6
  dry : Inport  Port=7
  drz : Inport  Port=8
  dly : Inport  Port=9
  dlz : Inport  Port=10
  Constant{,3,7,10} (4 alike) : Constant  Value=0
  Constant1 : Constant  Value=Mode_deflection_aileron
  Constant2 : Constant  Value=Mode_deflection_elevator
  Constant4 : Constant  Value=Mode_deflection_TVC_y
  Constant5 : Constant  Value=Mode_deflection_rudder
  Constant6 : Constant  Value=Mode_deflection_TVC_y
  Constant8 : Constant  Value=Mode_deflection_TVC_z
  Constant9 : Constant  Value=Mode_deflection_TVC_z
  Gain : Gain  Gain=-1
  Gain1 : Gain  Gain=-1
  Gain2 : Gain  Gain=-1
  Multiport Switch : MultiPortSwitch  DataPortOrder=Zero-based contiguous  Inputs=2  zeroidx=on  SaturateOnIntegerOverflow=off  InputSameDT=off
  Multiport Switch1 : MultiPortSwitch  DataPortOrder=Zero-based contiguous  Inputs=2  zeroidx=on  SaturateOnIntegerOverflow=off  InputSameDT=off
  Multiport Switch2 : MultiPortSwitch  DataPortOrder=Zero-based contiguous  DataPortForDefault=Additional data port  zeroidx=on  SaturateOnIntegerOverflow=off  InputSameDT=off
  Multiport Switch3 : MultiPortSwitch  DataPortOrder=Zero-based contiguous  Inputs=4  DataPortForDefault=Additional data port  zeroidx=on  SaturateOnIntegerOverflow=off  InputSameDT=off
  Multiport Switch4 : MultiPortSwitch  DataPortOrder=Zero-based contiguous  DataPortForDefault=Additional data port  zeroidx=on  SaturateOnIntegerOverflow=off  InputSameDT=off
  Multiport Switch5 : MultiPortSwitch  DataPortOrder=Zero-based contiguous  Inputs=4  DataPortForDefault=Additional data port  zeroidx=on  SaturateOnIntegerOverflow=off  InputSameDT=off
  Multiport Switch6 : MultiPortSwitch  DataPortOrder=Zero-based contiguous  DataPortForDefault=Additional data port  zeroidx=on  SaturateOnIntegerOverflow=off  InputSameDT=off
  right_aileron : Outport  VectorParamsAs1DForOutWhenUnconnected=off
  left_aileron : Outport  Port=2  VectorParamsAs1DForOutWhenUnconnected=off
  right_elevator : Outport  Port=3  VectorParamsAs1DForOutWhenUnconnected=off
  left_elevator : Outport  Port=4  VectorParamsAs1DForOutWhenUnconnected=off
  rudder : Outport  Port=5  VectorParamsAs1DForOutWhenUnconnected=off
  left_rudder : Outport  Port=6  VectorParamsAs1DForOutWhenUnconnected=off
  "TVC_ry " : Outport  Port=7  VectorParamsAs1DForOutWhenUnconnected=off
  TVC_rz : Outport  Port=8  VectorParamsAs1DForOutWhenUnconnected=off
  "TVC_ly " : Outport  Port=9  VectorParamsAs1DForOutWhenUnconnected=off
  "TVC_lz " : Outport  Port=10  VectorParamsAs1DForOutWhenUnconnected=off
  wires:
  Gain2/1 -> Multiport Switch3/5
  Gain1/1 -> Multiport Switch4/4
  Multiport Switch4/1 -> left_rudder/1
  Multiport Switch2/1 -> "TVC_lz "/1
  Constant3/1 -> Multiport Switch2/2
  drz/1 -> Multiport Switch6/3, Multiport Switch6/4, Multiport Switch6/5, Multiport Switch2/4
  Constant10/1 -> Multiport Switch6/2
  Multiport Switch6/1 -> TVC_rz/1
  Constant8/1 -> Multiport Switch2/1
  dlz/1 -> Multiport Switch2/3, Multiport Switch2/5
  Constant9/1 -> Multiport Switch6/1
  Multiport Switch5/1 -> "TVC_ry "/1
  Constant7/1 -> Multiport Switch5/2
  Constant6/1 -> Multiport Switch5/1
  Constant/1 -> Multiport Switch3/2
  dly/1 -> Multiport Switch3/6, Multiport Switch3/3
  Multiport Switch/1 -> left_aileron/1
  dre/1 -> right_elevator/1, Multiport Switch1/2
  dle/1 -> Multiport Switch1/3
  Multiport Switch1/1 -> left_elevator/1
  dla/1 -> Multiport Switch/3
  drr/1 -> Multiport Switch4/2, Gain1/1, rudder/1
  dry/1 -> Gain2/1, Multiport Switch3/4, Multiport Switch5/6, Multiport Switch5/5, Multiport Switch5/4, Multiport Switch5/3
  Constant5/1 -> Multiport Switch4/1
  dra/1 -> right_aileron/1, Gain/1
  Constant2/1 -> Multiport Switch1/1
  Constant4/1 -> Multiport Switch3/1
  Gain/1 -> Multiport Switch/2
  Constant1/1 -> Multiport Switch/1
  dlr/1 -> Multiport Switch4/3, Multiport Switch4/5
  Multiport Switch3/1 -> "TVC_ly "/1

== system Linearization2/F-16 Vehicle Systems Model/sysID_Onboard_Excitation_System/signal generator ==
  note: ROM記憶體的指標(Pointer)
  note: 唯讀記憶體，裡面存放波形
  isTurnOn : Inport
  Enable : Inport  Port=2
  sysID_isDone : Inport  Port=3
  Constant1 : Constant  Value=sysID_OBES.TVC_ry.amplitude
  Index Vector : MultiPortSwitch  Inputs=1  SaturateOnIntegerOverflow=off  InputSameDT=off
  Logical Operator1 : Logic  AllPortsSameDT=off  OutDataTypeStr=boolean
  Logical Operator3 : Logic  Operator=NOT  AllPortsSameDT=off  OutDataTypeStr=boolean
  Logical Operator4 : Logic  AllPortsSameDT=off  OutDataTypeStr=boolean
  Pause Counter : Subsystem  TreatAsAtomicUnit=on
  Product : Product
  ROM : Constant  Value=sysID_OBES.TVC_ry.wave
  TVC_ry_delay : Delay  DelayLength=sysID_OBES.TVC_ry.delay/sysID_OBES.Ts  SampleTime=sysID_OBES.Ts
  signal : Outport  OutputWhenDisabled=reset  InitialOutput=0
  isDone : Outport  Port=2
  wires:
  ROM/1 -> Index Vector/2
  Pause Counter/1(CountValue) -> Index Vector/1  "Pointer"
  Pause Counter/2(isCountDone) -> isDone/1
  Constant1/1 -> Product/1
  Index Vector/1 -> Product/2
  Product/1 -> signal/1
  Logical Operator3/1 -> Logical Operator4/2
  sysID_isDone/1 -> Logical Operator3/1  "isDone"
  TVC_ry_delay/1 -> Logical Operator4/1
  Enable/1 -> TVC_ry_delay/1  "isEnable"
  isTurnOn/1 -> Logical Operator1/1  "isTurnOn"
  Logical Operator4/1 -> Logical Operator1/2  "enableSignal"
  Logical Operator1/1 -> Pause Counter/Enable

== system Linearization2/F-16 Vehicle Systems Model/sysID_Onboard_Excitation_System/signal generator1 ==
  note: ROM記憶體的指標(Pointer)
  note: 唯讀記憶體，裡面存放波形
  isTurnOn : Inport
  Enable : Inport  Port=2
  sysID_isDone : Inport  Port=3
  Constant1 : Constant  Value=sysID_OBES.TVC_rz.amplitude
  Index Vector : MultiPortSwitch  Inputs=1  SaturateOnIntegerOverflow=off  InputSameDT=off
  Logical Operator1 : Logic  AllPortsSameDT=off  OutDataTypeStr=boolean
  Logical Operator3 : Logic  Operator=NOT  AllPortsSameDT=off  OutDataTypeStr=boolean
  Logical Operator4 : Logic  AllPortsSameDT=off  OutDataTypeStr=boolean
  Pause Counter : Subsystem  TreatAsAtomicUnit=on
  Product : Product
  ROM : Constant  Value=sysID_OBES.TVC_rz.wave
  TVC_rz_delay : Delay  DelayLength=sysID_OBES.TVC_rz.delay/sysID_OBES.Ts  SampleTime=sysID_OBES.Ts
  signal : Outport  OutputWhenDisabled=reset  InitialOutput=0
  isDone : Outport  Port=2
  wires:
  ROM/1 -> Index Vector/2
  Pause Counter/1(CountValue) -> Index Vector/1  "Pointer"
  Pause Counter/2(isCountDone) -> isDone/1
  Constant1/1 -> Product/1
  Index Vector/1 -> Product/2
  Product/1 -> signal/1
  Logical Operator3/1 -> Logical Operator4/2
  sysID_isDone/1 -> Logical Operator3/1  "isDone"
  TVC_rz_delay/1 -> Logical Operator4/1
  Enable/1 -> TVC_rz_delay/1  "isEnable"
  isTurnOn/1 -> Logical Operator1/1  "isTurnOn"
  Logical Operator4/1 -> Logical Operator1/2  "enableSignal"
  Logical Operator1/1 -> Pause Counter/Enable

== system Linearization2/F-16 Vehicle Systems Model/sysID_Onboard_Excitation_System/signal generator2 ==
  note: ROM記憶體的指標(Pointer)
  note: 唯讀記憶體，裡面存放波形
  isTurnOn : Inport
  Enable : Inport  Port=2
  sysID_isDone : Inport  Port=3
  Constant1 : Constant  Value=sysID_OBES.TVC_ly.amplitude
  Index Vector : MultiPortSwitch  Inputs=1  SaturateOnIntegerOverflow=off  InputSameDT=off
  Logical Operator1 : Logic  AllPortsSameDT=off  OutDataTypeStr=boolean
  Logical Operator3 : Logic  Operator=NOT  AllPortsSameDT=off  OutDataTypeStr=boolean
  Logical Operator4 : Logic  AllPortsSameDT=off  OutDataTypeStr=boolean
  Pause Counter : Subsystem  TreatAsAtomicUnit=on
  Product : Product
  ROM : Constant  Value=sysID_OBES.TVC_ly.wave
  TVC_ly_delay : Delay  DelayLength=sysID_OBES.TVC_ly.delay/sysID_OBES.Ts  SampleTime=sysID_OBES.Ts
  signal : Outport  OutputWhenDisabled=reset  InitialOutput=0
  isDone : Outport  Port=2
  wires:
  ROM/1 -> Index Vector/2
  Pause Counter/1(CountValue) -> Index Vector/1  "Pointer"
  Pause Counter/2(isCountDone) -> isDone/1
  Constant1/1 -> Product/1
  Index Vector/1 -> Product/2
  Product/1 -> signal/1
  Logical Operator3/1 -> Logical Operator4/2
  sysID_isDone/1 -> Logical Operator3/1  "isDone"
  TVC_ly_delay/1 -> Logical Operator4/1
  Enable/1 -> TVC_ly_delay/1  "isEnable"
  isTurnOn/1 -> Logical Operator1/1  "isTurnOn"
  Logical Operator4/1 -> Logical Operator1/2  "enableSignal"
  Logical Operator1/1 -> Pause Counter/Enable

== system Linearization2/F-16 Vehicle Systems Model/sysID_Onboard_Excitation_System/signal generator3 ==
  note: ROM記憶體的指標(Pointer)
  note: 唯讀記憶體，裡面存放波形
  isTurnOn : Inport
  Enable : Inport  Port=2
  sysID_isDone : Inport  Port=3
  Constant1 : Constant  Value=sysID_OBES.TVC_lz.amplitude
  Index Vector : MultiPortSwitch  Inputs=1  SaturateOnIntegerOverflow=off  InputSameDT=off
  Logical Operator1 : Logic  AllPortsSameDT=off  OutDataTypeStr=boolean
  Logical Operator3 : Logic  Operator=NOT  AllPortsSameDT=off  OutDataTypeStr=boolean
  Logical Operator4 : Logic  AllPortsSameDT=off  OutDataTypeStr=boolean
  Pause Counter : Subsystem  TreatAsAtomicUnit=on
  Product : Product
  ROM : Constant  Value=sysID_OBES.TVC_lz.wave
  TVC_lz_delay : Delay  DelayLength=sysID_OBES.TVC_lz.delay/sysID_OBES.Ts  SampleTime=sysID_OBES.Ts
  signal : Outport  OutputWhenDisabled=reset  InitialOutput=0
  isDone : Outport  Port=2
  wires:
  ROM/1 -> Index Vector/2
  Pause Counter/1(CountValue) -> Index Vector/1  "Pointer"
  Pause Counter/2(isCountDone) -> isDone/1
  Constant1/1 -> Product/1
  Index Vector/1 -> Product/2
  Product/1 -> signal/1
  Logical Operator3/1 -> Logical Operator4/2
  sysID_isDone/1 -> Logical Operator3/1  "isDone"
  TVC_lz_delay/1 -> Logical Operator4/1
  Enable/1 -> TVC_lz_delay/1  "isEnable"
  isTurnOn/1 -> Logical Operator1/1  "isTurnOn"
  Logical Operator4/1 -> Logical Operator1/2  "enableSignal"
  Logical Operator1/1 -> Pause Counter/Enable

== system Linearization2/F-16 Vehicle Systems Model/sysID_Onboard_Excitation_System/signal generator4 ==
  note: ROM記憶體的指標(Pointer)
  note: 唯讀記憶體，裡面存放波形
  isTurnOn : Inport
  Enable : Inport  Port=2
  sysID_isDone : Inport  Port=3
  Constant1 : Constant  Value=sysID_OBES.right_aileron.amplitude
  Index Vector : MultiPortSwitch  Inputs=1  SaturateOnIntegerOverflow=off  InputSameDT=off
  Logical Operator1 : Logic  AllPortsSameDT=off  OutDataTypeStr=boolean
  Logical Operator3 : Logic  Operator=NOT  AllPortsSameDT=off  OutDataTypeStr=boolean
  Logical Operator4 : Logic  AllPortsSameDT=off  OutDataTypeStr=boolean
  Pause Counter : Subsystem  TreatAsAtomicUnit=on
  Product : Product
  ROM : Constant  Value=sysID_OBES.right_aileron.wave
  right_aileron_delay : Delay  DelayLength=sysID_OBES.right_aileron.delay/sysID_OBES.Ts  SampleTime=sysID_OBES.Ts
  signal : Outport  OutputWhenDisabled=reset  InitialOutput=0
  isDone : Outport  Port=2
  wires:
  ROM/1 -> Index Vector/2
  Pause Counter/1(CountValue) -> Index Vector/1  "Pointer"
  Pause Counter/2(isCountDone) -> isDone/1
  Constant1/1 -> Product/1
  Index Vector/1 -> Product/2
  Product/1 -> signal/1
  Logical Operator3/1 -> Logical Operator4/2
  sysID_isDone/1 -> Logical Operator3/1  "isDone"
  right_aileron_delay/1 -> Logical Operator4/1
  Enable/1 -> right_aileron_delay/1  "isEnable"
  isTurnOn/1 -> Logical Operator1/1  "isTurnOn"
  Logical Operator4/1 -> Logical Operator1/2  "enableSignal"
  Logical Operator1/1 -> Pause Counter/Enable

== system Linearization2/F-16 Vehicle Systems Model/sysID_Onboard_Excitation_System/signal generator5 ==
  note: ROM記憶體的指標(Pointer)
  note: 唯讀記憶體，裡面存放波形
  isTurnOn : Inport
  Enable : Inport  Port=2
  sysID_isDone : Inport  Port=3
  Constant1 : Constant  Value=sysID_OBES.left_aileron.amplitude
  Index Vector : MultiPortSwitch  Inputs=1  SaturateOnIntegerOverflow=off  InputSameDT=off
  Logical Operator1 : Logic  AllPortsSameDT=off  OutDataTypeStr=boolean
  Logical Operator3 : Logic  Operator=NOT  AllPortsSameDT=off  OutDataTypeStr=boolean
  Logical Operator4 : Logic  AllPortsSameDT=off  OutDataTypeStr=boolean
  Pause Counter : Subsystem  TreatAsAtomicUnit=on
  Product : Product
  ROM : Constant  Value=sysID_OBES.left_aileron.wave
  left_aileron_delay : Delay  DelayLength=sysID_OBES.left_aileron.delay/sysID_OBES.Ts  SampleTime=sysID_OBES.Ts
  signal : Outport  OutputWhenDisabled=reset  InitialOutput=0
  isDone : Outport  Port=2
  wires:
  ROM/1 -> Index Vector/2
  Pause Counter/1(CountValue) -> Index Vector/1  "Pointer"
  Pause Counter/2(isCountDone) -> isDone/1
  Constant1/1 -> Product/1
  Index Vector/1 -> Product/2
  Product/1 -> signal/1
  Logical Operator3/1 -> Logical Operator4/2
  sysID_isDone/1 -> Logical Operator3/1  "isDone"
  left_aileron_delay/1 -> Logical Operator4/1
  Enable/1 -> left_aileron_delay/1  "isEnable"
  isTurnOn/1 -> Logical Operator1/1  "isTurnOn"
  Logical Operator4/1 -> Logical Operator1/2  "enableSignal"
  Logical Operator1/1 -> Pause Counter/Enable

== system Linearization2/F-16 Vehicle Systems Model/sysID_Onboard_Excitation_System/signal generator6 ==
  note: ROM記憶體的指標(Pointer)
  note: 唯讀記憶體，裡面存放波形
  isTurnOn : Inport
  Enable : Inport  Port=2
  sysID_isDone : Inport  Port=3
  Constant1 : Constant  Value=sysID_OBES.right_elevator.amplitude
  Index Vector : MultiPortSwitch  Inputs=1  SaturateOnIntegerOverflow=off  InputSameDT=off
  Logical Operator1 : Logic  AllPortsSameDT=off  OutDataTypeStr=boolean
  Logical Operator3 : Logic  Operator=NOT  AllPortsSameDT=off  OutDataTypeStr=boolean
  Logical Operator4 : Logic  AllPortsSameDT=off  OutDataTypeStr=boolean
  Pause Counter : Subsystem  TreatAsAtomicUnit=on
  Product : Product
  ROM : Constant  Value=sysID_OBES.right_elevator.wave
  right_elevator_delay : Delay  DelayLength=sysID_OBES.right_elevator.delay/sysID_OBES.Ts  SampleTime=sysID_OBES.Ts
  signal : Outport  OutputWhenDisabled=reset  InitialOutput=0
  isDone : Outport  Port=2
  wires:
  ROM/1 -> Index Vector/2
  Pause Counter/1(CountValue) -> Index Vector/1  "Pointer"
  Pause Counter/2(isCountDone) -> isDone/1
  Constant1/1 -> Product/1
  Index Vector/1 -> Product/2
  Product/1 -> signal/1
  Logical Operator3/1 -> Logical Operator4/2
  sysID_isDone/1 -> Logical Operator3/1  "isDone"
  right_elevator_delay/1 -> Logical Operator4/1
  Enable/1 -> right_elevator_delay/1  "isEnable"
  isTurnOn/1 -> Logical Operator1/1  "isTurnOn"
  Logical Operator4/1 -> Logical Operator1/2  "enableSignal"
  Logical Operator1/1 -> Pause Counter/Enable

== system Linearization2/F-16 Vehicle Systems Model/sysID_Onboard_Excitation_System/signal generator7 ==
  note: ROM記憶體的指標(Pointer)
  note: 唯讀記憶體，裡面存放波形
  isTurnOn : Inport
  Enable : Inport  Port=2
  sysID_isDone : Inport  Port=3
  Constant1 : Constant  Value=sysID_OBES.left_elevator.amplitude
  Index Vector : MultiPortSwitch  Inputs=1  SaturateOnIntegerOverflow=off  InputSameDT=off
  Logical Operator1 : Logic  AllPortsSameDT=off  OutDataTypeStr=boolean
  Logical Operator3 : Logic  Operator=NOT  AllPortsSameDT=off  OutDataTypeStr=boolean
  Logical Operator4 : Logic  AllPortsSameDT=off  OutDataTypeStr=boolean
  Pause Counter : Subsystem  TreatAsAtomicUnit=on
  Product : Product
  ROM : Constant  Value=sysID_OBES.left_elevator.wave
  left_elevator_delay : Delay  DelayLength=sysID_OBES.left_elevator.delay/sysID_OBES.Ts  SampleTime=sysID_OBES.Ts
  signal : Outport  OutputWhenDisabled=reset  InitialOutput=0
  isDone : Outport  Port=2
  wires:
  ROM/1 -> Index Vector/2
  Pause Counter/1(CountValue) -> Index Vector/1  "Pointer"
  Pause Counter/2(isCountDone) -> isDone/1
  Constant1/1 -> Product/1
  Index Vector/1 -> Product/2
  Product/1 -> signal/1
  Logical Operator3/1 -> Logical Operator4/2
  sysID_isDone/1 -> Logical Operator3/1  "isDone"
  left_elevator_delay/1 -> Logical Operator4/1
  Enable/1 -> left_elevator_delay/1  "isEnable"
  isTurnOn/1 -> Logical Operator1/1  "isTurnOn"
  Logical Operator4/1 -> Logical Operator1/2  "enableSignal"
  Logical Operator1/1 -> Pause Counter/Enable
